simulink model "Test3S150Board_HSMB"  (Simulink 6.4)
settings: Solver=ode45  SolverMode=SingleTasking  StartTime=0.0  StopTime=1000.0  FixedStep=1  RelTol=1e-3
InitFcn:
  | %% DSPBuilder Start
  | alt_dspbuilder_update_model(bdroot)
  | %% DSPBuilder End
undefined symbols (not defined in the file): Pin_AB24, Pin_AB25, Pin_AF31, Pin_AF32, Pin_C1, Pin_D1, Pin_D2, Pin_D3, Pin_E1, Pin_E2, Pin_F1, Pin_G1, Pin_G2, Pin_H1, Pin_H2, Pin_H3, Pin_H4, Pin_H5, Pin_H6, Pin_J1, Pin_J6, Pin_J7, Pin_K5, Pin_K6, Pin_K7, Pin_K8, Pin_L1, Pin_L2, Pin_L4, Pin_L5, Pin_L6, Pin_L7, Pin_L8, Pin_L9, Pin_M1, Pin_N1, Pin_N2, Pin_P1, Pin_P10, Pin_P11, Pin_P2, Pin_P3, Pin_P4, Pin_R1, Pin_R10, Pin_R3, Pin_R4, Pin_R6, Pin_R7, Pin_R9, Pin_T4, Pin_T5, Pin_T7, Pin_T8, Pin_T9, Pin_U6
libraries: allblocks_alteradspbuilder2 x49, Stratix_III_EP3SL150_alteradspbuilder2 x5
settings Model: Creator=lkong  LastModifiedBy=lkong
settings DataIOCC: SignalLoggingName=sigsOut
settings OptimizationCC: InlineInvariantSignals=on
settings DebuggingCC: SolverPrmCheckMsg=none  StrictBusMsg=None
settings HardwareCC: TargetUnknown=on
settings GRTTargetCC: ModelReferenceCompliant=off  MatFileLogging=off

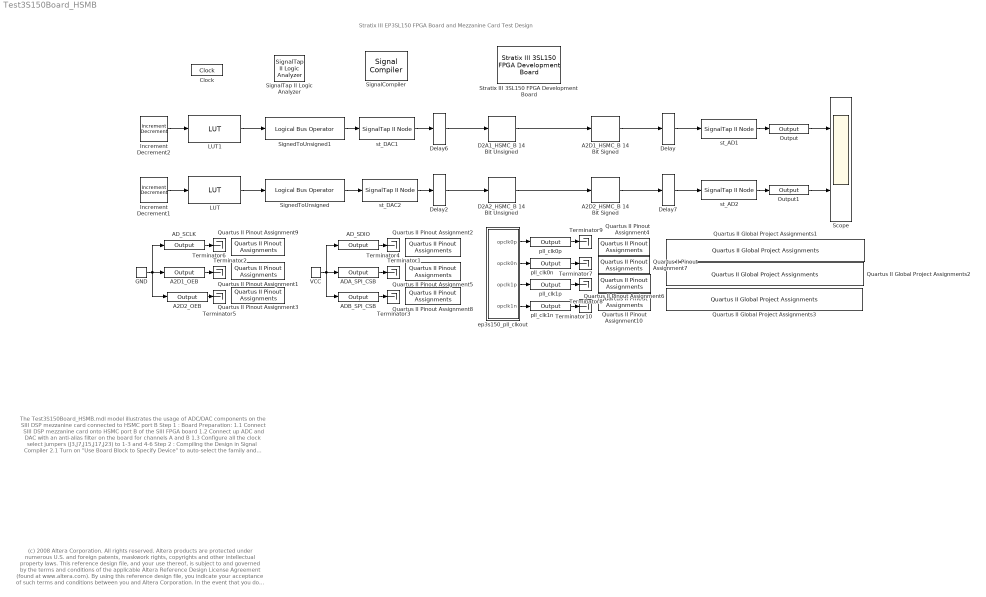
== system Test3S150Board_HSMB ==
  note: Stratix III EP3SL150 FPGA Board and Mezzanine Card Test Design
  note: (c) 2008 Altera Corporation. All rights reserved.  Altera products are protected under numerous U.S. and foreign patents, maskwork rights, copyrights and other intellectual property laws.
      | This reference design file, and your use thereof, is subject to and governed by the terms and conditions of the applicable Altera Reference Design License Agreement (found at www.altera.com).
      | By using this reference design file, you indicate your acceptance of such terms and conditions between you and Altera Corporation.
      | In the event that you do not agree with such terms and conditions, you may not use the reference design file and please promptly destroy any copies you have made.
      | This reference design file being provided on an "as-is" basis and as an accommodation and therefore all warranties, representations or guarantees of any kind (whether express, implied or statutory)
      | including, without limitation, warranties of merchantability, non-infringement, or fitness for a particular purpose, are specifically disclaimed.
      | By making this reference design file available, Altera expressly does not recommend, suggest or require that this reference design file be used in combination with any other product not provided by Altera
  note: The Test3S150Board_HSMB.mdl model illustrates the usage of ADC/DAC components on the SIII DSP mezzanine card connected to HSMC port B
      |
      | Step 1 : Board Preparation:
      |                1.1 Connect SIII DSP mezzanine card onto HSMC port B of the SIII FPGA board
      |                1.2 Connect up ADC and DAC with an anti-alias filter on the board for channels A and B
      |                1.3 Configure all the clock select jumpers (J3,J7,J15,J17,J23) to 1-3 and 4-6
      | Step 2 : Compiling the Design in Signal Compiler
      |                2.1 Turn on "Use Board Block to Specify Device" to auto-select the family and device
      |                2.2 Click "Compile" to compile the design through the Quartus II software and create a .sof file
      |                2.3 Click "Scan Jtag" to select a download cable and device
      |                2.4 Click "Program" to download the .sof file onto the FPGA device
      | Step 3 : Running SignalTap II Logic Analyzer
      |                3.1 Click "Scan Jtag" to select a download cable and device
      |                3.2 Click "Acquire" to obtain data for embedded SignalTap II nodes
  A2D1_HSMC_B 14 Bit Signed : Stratix_III_EP3SL150_alteradspbuilder2/A2D1_HSMC_B 14 Bit Signed  iofile=d:\ws80\workspace\Documentation\DesignExamples\Demos\Board\StratixIII_DSPBoard_3S150\tb_Test3S150Board_HSMB\Test3S150Board%5FHSMB_A2D1%5FHSMC%5FB+14+Bit+Signed.salt  externalType=Inferred  SpecifyClock=off  location=Pin_R6,Pin_R7,Pin_R9,Pin_R10,Pin_T4,Pin_T5,Pin_U6,Pin_T7,Pin_T8,Pin_T9,Pin_P10,Pin_P11,Pin_AF32,Pin_AB24
  A2D1_OEB : allblocks_alteradspbuilder2/Output  iofile=d:\ws80\workspace\Documentation\DesignExamples\Demos\Board\StratixIII_DSPBoard_3S150\tb_Test3S150Board_HSMB\Test3S150Board%5FHSMB_A2D1%5FOEB.capture  BusType=Single Bit  bwl=1  bwr=0  externalType=Inferred  PORTTYPE=Output  allowFloatingPointOverride=on  logOutputs=off
  A2D2_HSMC_B 14 Bit Signed : Stratix_III_EP3SL150_alteradspbuilder2/A2D2_HSMC_B 14 Bit Signed  iofile=d:\ws80\workspace\Documentation\DesignExamples\Demos\Board\StratixIII_DSPBoard_3S150\tb_Test3S150Board_HSMB\Test3S150Board%5FHSMB_A2D2%5FHSMC%5FB+14+Bit+Signed.salt  externalType=Inferred  SpecifyClock=off  location=Pin_L1,Pin_L2,Pin_N1,Pin_M1,Pin_P1,Pin_N2,Pin_R1,Pin_P2,Pin_P3,Pin_P4,Pin_R3,Pin_R4,Pin_AF31,Pin_AB25
  A2D2_OEB : allblocks_alteradspbuilder2/Output  iofile=d:\ws80\workspace\Documentation\DesignExamples\Demos\Board\StratixIII_DSPBoard_3S150\tb_Test3S150Board_HSMB\Test3S150Board%5FHSMB_A2D2%5FOEB.capture  BusType=Single Bit  bwl=1  bwr=0  externalType=Inferred  PORTTYPE=Output  allowFloatingPointOverride=on  logOutputs=off
  ADA_SPI_CSB : allblocks_alteradspbuilder2/Output  iofile=d:\ws80\workspace\Documentation\DesignExamples\Demos\Board\StratixIII_DSPBoard_3S150\tb_Test3S150Board_HSMB\Test3S150Board%5FHSMB_ADA%5FSPI%5FCSB.capture  BusType=Single Bit  bwl=1  bwr=0  externalType=Inferred  PORTTYPE=Output  allowFloatingPointOverride=on  logOutputs=off
  ADB_SPI_CSB : allblocks_alteradspbuilder2/Output  iofile=d:\ws80\workspace\Documentation\DesignExamples\Demos\Board\StratixIII_DSPBoard_3S150\tb_Test3S150Board_HSMB\Test3S150Board%5FHSMB_ADB%5FSPI%5FCSB.capture  BusType=Single Bit  bwl=1  bwr=0  externalType=Inferred  PORTTYPE=Output  allowFloatingPointOverride=on  logOutputs=off
  AD_SCLK : allblocks_alteradspbuilder2/Output  iofile=d:\ws80\workspace\Documentation\DesignExamples\Demos\Board\StratixIII_DSPBoard_3S150\tb_Test3S150Board_HSMB\Test3S150Board%5FHSMB_AD%5FSCLK.capture  BusType=Single Bit  bwl=1  bwr=0  externalType=Inferred  PORTTYPE=Output  allowFloatingPointOverride=on  logOutputs=off
  AD_SDIO : allblocks_alteradspbuilder2/Output  iofile=d:\ws80\workspace\Documentation\DesignExamples\Demos\Board\StratixIII_DSPBoard_3S150\tb_Test3S150Board_HSMB\Test3S150Board%5FHSMB_AD%5FSDIO.capture  BusType=Single Bit  bwl=1  bwr=0  externalType=Inferred  PORTTYPE=Output  allowFloatingPointOverride=on  logOutputs=off
  Clock : allblocks_alteradspbuilder2/Clock  ClockPeriod=20  ClockPeriodUnit=ns  SampleTime=1  SimulationStartCycle=5  PhaseOffset=0  Reset=aclr  ResetType=Active Low  Export=off
  D2A1_HSMC_B 14 Bit Unsigned : Stratix_III_EP3SL150_alteradspbuilder2/D2A1_HSMC_B 14 Bit Unsigned  iofile=d:\ws80\workspace\Documentation\DesignExamples\Demos\Board\StratixIII_DSPBoard_3S150\tb_Test3S150Board_HSMB\Test3S150Board%5FHSMB_D2A1%5FHSMC%5FB+14+Bit+Unsigned.capture  externalType=Inferred  location=Pin_L8,Pin_L9,Pin_K7,Pin_K8,Pin_H5,Pin_H6,Pin_J6,Pin_J7,Pin_K5,Pin_K6,Pin_L4,Pin_L5,Pin_L6,Pin_L7
  D2A2_HSMC_B 14 Bit Unsigned : Stratix_III_EP3SL150_alteradspbuilder2/D2A2_HSMC_B 14 Bit Unsigned  iofile=d:\ws80\workspace\Documentation\DesignExamples\Demos\Board\StratixIII_DSPBoard_3S150\tb_Test3S150Board_HSMB\Test3S150Board%5FHSMB_D2A2%5FHSMC%5FB+14+Bit+Unsigned.capture  externalType=Inferred  location=Pin_D2,Pin_D3,Pin_D1,Pin_C1,Pin_E1,Pin_E2,Pin_H3,Pin_H4,Pin_G1,Pin_F1,Pin_H1,Pin_G2,Pin_J1,Pin_H2
  Delay : allblocks_alteradspbuilder2/Delay  pipeline=1  pipeline_display=1  ClockPhase=1  use_ena=off  use_sclr=off  allowFloatingPointOverride=on  logOutputs=off  logFile=d:\ws80\workspace\Documentation\DesignExamples\Demos\Board\StratixIII_DSPBoard_3S150\tb_Test3S150Board_HSMB\Test3S150Board%5FHSMB_Delay.fixedpointlog  use_init=off  reset_value=1
  Delay2 : allblocks_alteradspbuilder2/Delay  pipeline=1  pipeline_display=1  ClockPhase=1  use_ena=off  use_sclr=off  allowFloatingPointOverride=on  logOutputs=off  logFile=d:\ws80\workspace\Documentation\DesignExamples\Demos\Board\StratixIII_DSPBoard_3S150\tb_Test3S150Board_HSMB\Test3S150Board%5FHSMB_Delay2.fixedpointlog  use_init=off  reset_value=1
  Delay6 : allblocks_alteradspbuilder2/Delay  pipeline=1  pipeline_display=1  ClockPhase=1  use_ena=off  use_sclr=off  allowFloatingPointOverride=on  logOutputs=off  logFile=d:\ws80\workspace\Documentation\DesignExamples\Demos\Board\StratixIII_DSPBoard_3S150\tb_Test3S150Board_HSMB\Test3S150Board%5FHSMB_Delay6.fixedpointlog  use_init=off  reset_value=1
  Delay7 : allblocks_alteradspbuilder2/Delay  pipeline=1  pipeline_display=1  ClockPhase=1  use_ena=off  use_sclr=off  allowFloatingPointOverride=on  logOutputs=off  logFile=d:\ws80\workspace\Documentation\DesignExamples\Demos\Board\StratixIII_DSPBoard_3S150\tb_Test3S150Board_HSMB\Test3S150Board%5FHSMB_Delay7.fixedpointlog  use_init=off  reset_value=1
  GND : allblocks_alteradspbuilder2/GND  SpecifyClock=off
  Increment Decrement1 : allblocks_alteradspbuilder2/Increment Decrement  BusType=Unsigned Integer  bwl=7  bwr=0  SpecifyClock=off  clr_value=0  direction=Increment  phase_selection=1  use_ena=off  use_sclr=off  pipeline_display=1
  Increment Decrement2 : allblocks_alteradspbuilder2/Increment Decrement  BusType=Unsigned Integer  bwl=7  bwr=0  SpecifyClock=off  clr_value=0  direction=Increment  phase_selection=1  use_ena=off  use_sclr=off  pipeline_display=1
  LUT : allblocks_alteradspbuilder2/LUT  addr_width=7  BusType=Signed Integer  bwl=14  bwr=0  init_array=8191*sin( [0:2*pi/(2^7):2*pi] )  allowFloatingPointOverride=on  logOutputs=off  logFile=d:\ws80\workspace\Documentation\DesignExamples\Demos\Board\StratixIII_DSPBoard_3S150\tb_Test3S150Board_HSMB\Test3S150Board%5FHSMB_LUT.fixedpointlog  use_ena=off  reg_data=on  use_lpm=on  reg_addr=on  ram_type=AUTO  pipeline_display=2
  LUT1 : allblocks_alteradspbuilder2/LUT  addr_width=7  BusType=Signed Integer  bwl=14  bwr=0  init_array=8191*sin( [0:2*pi/(2^7):2*pi] )  allowFloatingPointOverride=on  logOutputs=off  logFile=d:\ws80\workspace\Documentation\DesignExamples\Demos\Board\StratixIII_DSPBoard_3S150\tb_Test3S150Board_HSMB\Test3S150Board%5FHSMB_LUT1.fixedpointlog  use_ena=off  reg_data=on  use_lpm=on  reg_addr=on  ram_type=AUTO  pipeline_display=2
  Output : allblocks_alteradspbuilder2/Output  iofile=d:\ws80\workspace\Documentation\DesignExamples\Demos\Board\StratixIII_DSPBoard_3S150\tb_Test3S150Board_HSMB\Test3S150Board%5FHSMB_Output.capture  BusType=Signed Integer  bwl=14  bwr=0  externalType=Inferred  PORTTYPE=Output  allowFloatingPointOverride=on  logOutputs=off
  Output1 : allblocks_alteradspbuilder2/Output  iofile=d:\ws80\workspace\Documentation\DesignExamples\Demos\Board\StratixIII_DSPBoard_3S150\tb_Test3S150Board_HSMB\Test3S150Board%5FHSMB_Output1.capture  BusType=Signed Integer  bwl=14  bwr=0  externalType=Inferred  PORTTYPE=Output  allowFloatingPointOverride=on  logOutputs=off
  Quartus II Global Project Assignments1 : allblocks_alteradspbuilder2/Quartus II Global Project Assignments  QuartusIIAssignmentName=RESERVE_DATA1_AFTER_CONFIGURATION  QuartusIIAssignmentValue="\"USE AS REGULAR IO\""
  Quartus II Global Project Assignments2 : allblocks_alteradspbuilder2/Quartus II Global Project Assignments  QuartusIIAssignmentName=RESERVE_NCEO_AFTER_CONFIGURATION  QuartusIIAssignmentValue="\"USE AS REGULAR IO\""
  Quartus II Global Project Assignments3 : allblocks_alteradspbuilder2/Quartus II Global Project Assignments  QuartusIIAssignmentName=RESERVE_DCLK_AFTER_CONFIGURATION  QuartusIIAssignmentValue="\"USE AS REGULAR IO\""
  Quartus II Pinout Assignment1 : allblocks_alteradspbuilder2/Quartus II Pinout Assignments  QuartusIIAssignmentName=A2D1_OEB  QuartusIIAssignmentValue=Pin_N8
  Quartus II Pinout Assignment10 : allblocks_alteradspbuilder2/Quartus II Pinout Assignments  QuartusIIAssignmentName=pll_clk1n  QuartusIIAssignmentValue=Pin_T11
  Quartus II Pinout Assignment2 : allblocks_alteradspbuilder2/Quartus II Pinout Assignments  QuartusIIAssignmentName=AD_SDIO  QuartusIIAssignmentValue=Pin_M6
  Quartus II Pinout Assignment3 : allblocks_alteradspbuilder2/Quartus II Pinout Assignments  QuartusIIAssignmentName=A2D2_OEB  QuartusIIAssignmentValue=Pin_K3
  Quartus II Pinout Assignment4 : allblocks_alteradspbuilder2/Quartus II Pinout Assignments  QuartusIIAssignmentName=pll_clk0p  QuartusIIAssignmentValue=Pin_P6
  Quartus II Pinout Assignment5 : allblocks_alteradspbuilder2/Quartus II Pinout Assignments  QuartusIIAssignmentName=ADA_SPI_CSB  QuartusIIAssignmentValue=Pin_M7
  Quartus II Pinout Assignment6 : allblocks_alteradspbuilder2/Quartus II Pinout Assignments  QuartusIIAssignmentName=pll_clk1p  QuartusIIAssignmentValue=Pin_R12
  Quartus II Pinout Assignment7 : allblocks_alteradspbuilder2/Quartus II Pinout Assignments  QuartusIIAssignmentName=pll_clk0n  QuartusIIAssignmentValue=Pin_P5
  Quartus II Pinout Assignment8 : allblocks_alteradspbuilder2/Quartus II Pinout Assignments  QuartusIIAssignmentName=ADB_SPI_CSB  QuartusIIAssignmentValue=Pin_J4
  Quartus II Pinout Assignment9 : allblocks_alteradspbuilder2/Quartus II Pinout Assignments  QuartusIIAssignmentName=AD_SCLK  QuartusIIAssignmentValue=Pin_J3
  Scope : Scope  NumInputPorts=2
      settings: YMin=-5~-5  YMax=5~5  SampleInput=on
  SignalCompiler : allblocks_alteradspbuilder2/Signal Compiler  DeviceFamily=Stratix III  DeviceName=EP3SL150F1152C4  EnableSignalTap=on  SignalTapDepth=512  UseBoardBlock=on  StpUseDefaultClock=on  StpClock=Clock  ExportDir=D:\MATLAB\R2006a\work
  SignalTap II Logic Analyzer : allblocks_alteradspbuilder2/SignalTap II Logic Analyzer
  SignedToUnsigned : allblocks_alteradspbuilder2/Logical Bus Operator  BusType=Unsigned Integer  bwl=14  bwr=0  LogicalOp_text=XOR  mask_value_num=8192  shift_amount=3  force_sign_ext=off  pipeline_display=0
  SignedToUnsigned1 : allblocks_alteradspbuilder2/Logical Bus Operator  BusType=Unsigned Integer  bwl=14  bwr=0  LogicalOp_text=XOR  mask_value_num=8192  shift_amount=3  force_sign_ext=off  pipeline_display=0
  "Stratix III 3SL150 FPGA Development Board " : Stratix_III_EP3SL150_alteradspbuilder2/Stratix III 3SL150 FPGA Development Board   ClockPinIn=Pin_T33  GlobalResetPin=PIN_AP5  device=EP3SL150F1152C4
  Terminator{1..10} (10 alike) : Terminator
  VCC : allblocks_alteradspbuilder2/VCC  SpecifyClock=off
  ep3s150_pll_clkout : Subsystem
      mask Type: SubSystem AlteraBlockSet
  pll_clk0n : allblocks_alteradspbuilder2/Output  iofile=d:\ws80\workspace\Documentation\DesignExamples\Demos\Board\StratixIII_DSPBoard_3S150\tb_Test3S150Board_HSMB\Test3S150Board%5FHSMB_pll%5Fclk0n.capture  BusType=Single Bit  bwl=1  bwr=0  externalType=Inferred  PORTTYPE=Output  allowFloatingPointOverride=on  logOutputs=off
  pll_clk0p : allblocks_alteradspbuilder2/Output  iofile=d:\ws80\workspace\Documentation\DesignExamples\Demos\Board\StratixIII_DSPBoard_3S150\tb_Test3S150Board_HSMB\Test3S150Board%5FHSMB_pll%5Fclk0p.capture  BusType=Single Bit  bwl=1  bwr=0  externalType=Inferred  PORTTYPE=Output  allowFloatingPointOverride=on  logOutputs=off
  pll_clk1n : allblocks_alteradspbuilder2/Output  iofile=d:\ws80\workspace\Documentation\DesignExamples\Demos\Board\StratixIII_DSPBoard_3S150\tb_Test3S150Board_HSMB\Test3S150Board%5FHSMB_pll%5Fclk1n.capture  BusType=Single Bit  bwl=1  bwr=0  externalType=Inferred  PORTTYPE=Output  allowFloatingPointOverride=on  logOutputs=off
  pll_clk1p : allblocks_alteradspbuilder2/Output  iofile=d:\ws80\workspace\Documentation\DesignExamples\Demos\Board\StratixIII_DSPBoard_3S150\tb_Test3S150Board_HSMB\Test3S150Board%5FHSMB_pll%5Fclk1p.capture  BusType=Single Bit  bwl=1  bwr=0  externalType=Inferred  PORTTYPE=Output  allowFloatingPointOverride=on  logOutputs=off
  st_AD1 : allblocks_alteradspbuilder2/SignalTap II Node  id=0
  st_AD2 : allblocks_alteradspbuilder2/SignalTap II Node  id=1
  st_DAC1 : allblocks_alteradspbuilder2/SignalTap II Node  id=2
  st_DAC2 : allblocks_alteradspbuilder2/SignalTap II Node  id=3
  wires:
  SignedToUnsigned1/1 -> st_DAC1/1
  Delay/1 -> st_AD1/1
  Delay6/1 -> D2A1_HSMC_B 14 Bit Unsigned/1
  st_DAC1/1 -> Delay6/1
  D2A1_HSMC_B 14 Bit Unsigned/1 -> A2D1_HSMC_B 14 Bit Signed/1
  LUT/1 -> SignedToUnsigned/1
  SignedToUnsigned/1 -> st_DAC2/1
  Increment Decrement1/1 -> LUT/1
  Delay2/1 -> D2A2_HSMC_B 14 Bit Unsigned/1
  st_DAC2/1 -> Delay2/1
  D2A2_HSMC_B 14 Bit Unsigned/1 -> A2D2_HSMC_B 14 Bit Signed/1
  A2D1_HSMC_B 14 Bit Signed/1 -> Delay/1
  A2D2_HSMC_B 14 Bit Signed/1 -> Delay7/1
  Delay7/1 -> st_AD2/1
  st_AD1/1 -> Output/1
  st_AD2/1 -> Output1/1
  Output/1 -> Scope/1
  Output1/1 -> Scope/2
  LUT1/1 -> SignedToUnsigned1/1
  Increment Decrement2/1 -> LUT1/1
  A2D1_OEB/1 -> Terminator2/1
  A2D2_OEB/1 -> Terminator5/1
  GND/1 -> A2D2_OEB/1, A2D1_OEB/1, AD_SCLK/1
  ADA_SPI_CSB/1 -> Terminator1/1
  ADB_SPI_CSB/1 -> Terminator3/1
  VCC/1 -> ADB_SPI_CSB/1, ADA_SPI_CSB/1, AD_SDIO/1
  AD_SDIO/1 -> Terminator4/1
  AD_SCLK/1 -> Terminator6/1
  ep3s150_pll_clkout/1(opclk0p) -> pll_clk0p/1
  ep3s150_pll_clkout/2(opclk0n) -> pll_clk0n/1
  ep3s150_pll_clkout/3(opclk1p) -> pll_clk1p/1
  ep3s150_pll_clkout/4(opclk1n) -> pll_clk1n/1
  pll_clk0p/1 -> Terminator9/1
  pll_clk0n/1 -> Terminator7/1
  pll_clk1p/1 -> Terminator8/1
  pll_clk1n/1 -> Terminator10/1

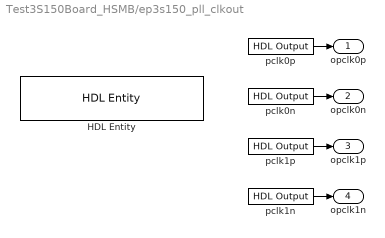
== system Test3S150Board_HSMB/ep3s150_pll_clkout ==
  HDL Entity : allblocks_alteradspbuilder2/HDL Entity  HDLFile=ep3s150_pll_clkout.vhd  clockname=clkin_50  useSubsystemPortName=off
  pclk0n : allblocks_alteradspbuilder2/HDL Output  BusType=Single Bit  bwl=1  bwr=0  externalType=Inferred
  pclk0p : allblocks_alteradspbuilder2/HDL Output  BusType=Single Bit  bwl=1  bwr=0  externalType=Inferred
  pclk1n : allblocks_alteradspbuilder2/HDL Output  BusType=Single Bit  bwl=1  bwr=0  externalType=Inferred
  pclk1p : allblocks_alteradspbuilder2/HDL Output  BusType=Single Bit  bwl=1  bwr=0  externalType=Inferred
  opclk0p : Outport
  opclk0n : Outport  Port=2
  opclk1p : Outport  Port=3
  opclk1n : Outport  Port=4
  wires:
  pclk0p/1 -> opclk0p/1
  pclk0n/1 -> opclk0n/1
  pclk1p/1 -> opclk1p/1
  pclk1n/1 -> opclk1n/1
